simulink model "dlqr_nonlinear_model"  (R2017a)
settings: Solver=ode5  StartTime=0.0  StopTime=7  FixedStep=0.0056  RelTol=1e-3
StartFcn:
  | global P xhat
  | P=diag([0.02 0.02 0]);
  | xhat=[1.25 0.81 1.35]';
values from neighbouring files (symbols this model uses):
  GAMAin = 100    [model_params.m]
  Ks = 0.012    [model_params.m]
  MUmax = 0.55    [model_params.m]
  T0 = 0.0056    [dlqr_reg.m]    (also in model_params.m)
  Ysx = 0.5    [model_params.m]
undefined symbols (not defined in the file or in its folder): DiscIntNeverNeededParam, K1
libraries: cstblocks x1
settings Model: Creator=user  LastModifiedBy=user

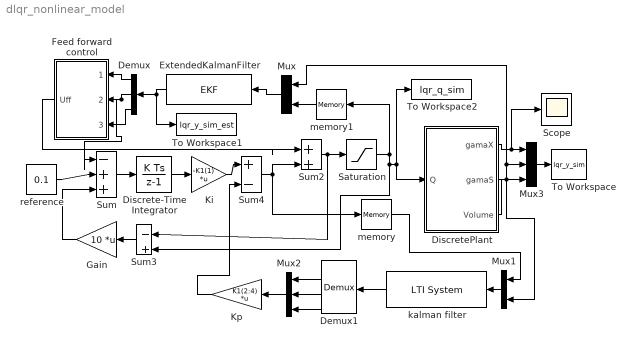
== system dlqr_nonlinear_model ==
  Demux : Demux  Outputs=3
  Demux1 : Demux
  Discrete-Time Integrator : DiscreteIntegrator  InitialConditionSetting=State (most efficient)  SampleTime=-1  ICPrevOutput=DiscIntNeverNeededParam  ICPrevScaledInput=DiscIntNeverNeededParam
  DiscretePlant : Subsystem
  ExtendedKalmanFilter : MATLABFcn  MATLABFcn=EKF  OutputDimensions=3  Output1D=off
  Feed forward control : Subsystem
  Gain : Gain  Gain=10  Multiplication=Matrix(K*u)
  Ki : Gain  Gain=-K1(1)  Multiplication=Matrix(K*u)
  Kp : Gain  Gain=K1(2:4)  Multiplication=Matrix(K*u)
  Mux : Mux  Inputs=2
  Mux1 : Mux  Inputs=2
  Mux2 : Mux  Inputs=3
  Mux3 : Mux  Inputs=3
  Saturation : Saturate  UpperLimit=1  LowerLimit=0
  Scope : Scope
  Sum : Sum  Inputs=|-++
  Sum2 : Sum  Inputs=|++
  Sum3 : Sum  Inputs=|-+
  Sum4 : Sum  Inputs=|+-
  To Workspace : ToWorkspace  VariableName=lqr_y_sim  SampleTime=-1
  To Workspace1 : ToWorkspace  VariableName=lqr_y_sim_est  SampleTime=-1
  To Workspace2 : ToWorkspace  VariableName=lqr_q_sim  SampleTime=-1
  "kalman filter " : cstblocks/LTI System  sys=Kal  IC=0
  memory : Memory
  memory1 : Memory
  reference : Constant  Value=0.1
  wires:
  ExtendedKalmanFilter/1 -> To Workspace1/1, Demux/1
  Mux/1 -> ExtendedKalmanFilter/1
  Sum/1 -> Discrete-Time Integrator/1
  Discrete-Time Integrator/1 -> Ki/1
  Ki/1 -> Sum4/1
  Sum4/1 -> Sum2/2, memory/1
  Feed forward control/1(Uff) -> Sum2/1
  Sum2/1 -> Sum3/1, Saturation/1
  Demux/1 -> Feed forward control/1(GAMAx)
  Demux/2 -> Sum/1, Feed forward control/2(GAMAs)
  Demux/3 -> Feed forward control/3(Volume)
  Mux1/1 -> "kalman filter "/1
  DiscretePlant/2(gamaS) -> Mux3/2, Mux/1, Mux1/2
  Mux2/1 -> Kp/1
  Demux1/4 -> Mux2/3
  Demux1/3 -> Mux2/2
  Demux1/2 -> Mux2/1
  "kalman filter "/1 -> Demux1/1
  Kp/1 -> Sum4/2
  Saturation/1 -> Sum3/2, DiscretePlant/1(Q), To Workspace2/1, memory1/1
  memory/1 -> Mux1/1
  Sum3/1 -> Gain/1
  reference/1 -> Sum/2
  Gain/1 -> Sum/3
  memory1/1 -> Mux/2
  DiscretePlant/3(Volume) -> Mux3/3
  Mux3/1 -> To Workspace/1
  DiscretePlant/1(gamaX) -> Scope/1, Mux3/1

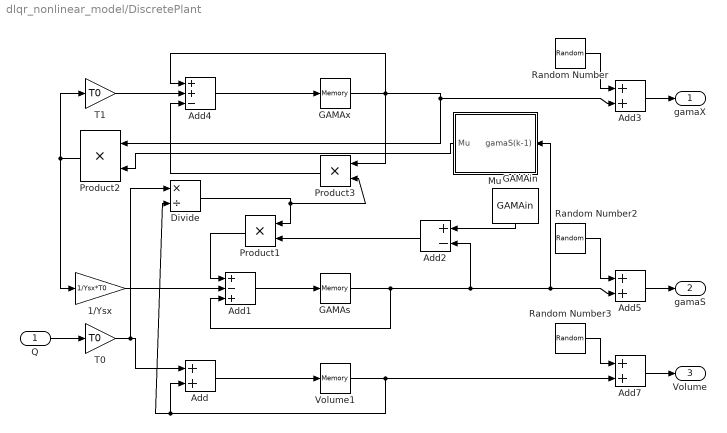
== system dlqr_nonlinear_model/DiscretePlant ==
  Q : Inport
  1/Ysx : Gain  Gain=1/Ysx*T0
  Add{,3,5,7} (4 alike) : Sum
  Add1 : Sum  Inputs=+-+
  Add2 : Sum  Inputs=+-
  Add4 : Sum  Inputs=++-
  Divide : Product  Inputs=*/
  GAMAin : Constant  Value=GAMAin
  GAMAs : Memory  X0=0.81
  GAMAx : Memory  X0=1.25
  Mu : Subsystem
  Product1 : Product  RndMeth=Zero
  Product2 : Product  RndMeth=Zero
  Product3 : Product  RndMeth=Zero
  Random Number : RandomNumber  Variance=0.0025  Seed=34645  SampleTime=0.0056
  Random Number2 : RandomNumber  Variance=0.0001  Seed=454645  SampleTime=0.0056
  Random Number3 : RandomNumber  Variance=0.0001  Seed=4546  SampleTime=0.0056
  T0 : Gain  Gain=T0
  T1 : Gain  Gain=T0
  Volume1 : Memory  X0=1.35
  gamaX : Outport
  gamaS : Outport  Port=2
  Volume : Outport  Port=3
  wires:
  Product1/1 -> Add1/1
  Add2/1 -> Product1/2
  GAMAin/1 -> Add2/1
  1/Ysx/1 -> Add1/2
  Product2/1 -> 1/Ysx/1, T1/1
  Product3/1 -> Add4/3
  Add1/1 -> GAMAs/1
  Add4/1 -> GAMAx/1
  Mu/1(Mu) -> Product2/2
  GAMAs/1 -> Add2/2, Mu/1(gamaS(k-1)), Add5/2, Add1/3
  GAMAx/1 -> Product3/1, Add4/1, Product2/1, Add3/2
  Add/1 -> Volume1/1
  Volume1/1 -> Divide/2, Add/2, Add7/2
  T0/1 -> Add/1, Divide/1
  Divide/1 -> Product1/1, Product3/2
  T1/1 -> Add4/2
  Add3/1 -> gamaX/1
  Add5/1 -> gamaS/1
  Q/1 -> T0/1
  Add7/1 -> Volume/1
  Random Number2/1 -> Add5/1
  Random Number/1 -> Add3/1
  Random Number3/1 -> Add7/1

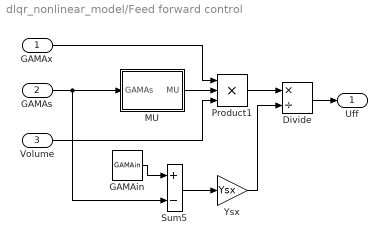
== system dlqr_nonlinear_model/Feed forward control ==
  GAMAx : Inport
  GAMAs : Inport  Port=2
  Volume : Inport  Port=3
  Divide : Product  Inputs=*/
  GAMAin : Constant  Value=GAMAin
  MU : Subsystem
  Product1 : Product  Inputs=3  RndMeth=Zero
  Sum5 : Sum  Inputs=+-
  Ysx : Gain  Gain=Ysx
  Uff : Outport
  wires:
  GAMAs/1 -> MU/1(GAMAs), Sum5/2
  GAMAx/1 -> Product1/1
  MU/1(MU) -> Product1/2
  Volume/1 -> Product1/3
  Sum5/1 -> Ysx/1
  GAMAin/1 -> Sum5/1
  Product1/1 -> Divide/1
  Ysx/1 -> Divide/2
  Divide/1 -> Uff/1

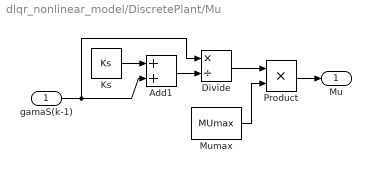
== system dlqr_nonlinear_model/DiscretePlant/Mu ==
  gamaS(k-1) : Inport
  Add1 : Sum
  Divide : Product  Inputs=*/
  Ks : Constant  Value=Ks
  Mumax : Constant  Value=MUmax
  Product : Product  RndMeth=Zero
  Mu : Outport
  wires:
  Ks/1 -> Add1/1
  Add1/1 -> Divide/2
  Divide/1 -> Product/1
  Mumax/1 -> Product/2
  Product/1 -> Mu/1
  gamaS(k-1)/1 -> Add1/2, Divide/1

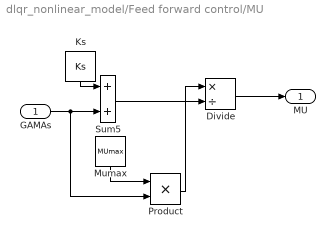
== system dlqr_nonlinear_model/Feed forward control/MU ==
  GAMAs : Inport
  Divide : Product  Inputs=*/
  Ks : Constant  Value=Ks
  Mumax : Constant  Value=MUmax
  Product : Product  RndMeth=Zero
  Sum5 : Sum
  MU : Outport
  wires:
  Product/1 -> Divide/1
  Mumax/1 -> Product/1
  Sum5/1 -> Divide/2
  GAMAs/1 -> Sum5/2, Product/2
  Ks/1 -> Sum5/1
  Divide/1 -> MU/1
